simulink model "generic_IsaacV3"  (R2015a)
settings: Solver=ode3  StartTime=0.0  StopTime=inf  FixedStep=0.001  RelTol=1e-3
values from neighbouring files (symbols this model uses):
  coast_domain = 0.1    [LoadVar.m]
  DifferentialFactor = 0.5    [LoadVar.m]
  g = 9.81    [LoadVar.m]
  GearRatio = 10.364    [LoadVar.m]
  Gr = 10.32    [LoadVar.m]
  Lf = 0.78    [LoadVar.m]
  Lr = 0.745    [LoadVar.m]
  M = 265    [LoadVar.m]
  max_coast_Nm = 0    [LoadVar.m]
  MaxSteeringAngle = 24.635    [LoadVar.m]
  mu_max = 1.5    [LoadVar.m]
  ped_max_limiet = 1    [LoadVar.m]
  pedal_position_maxacc = 0.9    [LoadVar.m]
  Reff = 0.2325    [LoadVar.m]
  regen_activation_kph = 15    [LoadVar.m]
  slewbreak_domain = 0.15    [LoadVar.m]
  Sr = 0.6    [LoadVar.m]
  T_max_Nm = 40    [LoadVar.m]
  T_min_Nm = -15    [LoadVar.m]
  TireRadius = 0.4572/2    (= 0.2286)    [LoadVar.m]
  Tmax = 40    [LoadVar.m]
  TrackLength = 1.534    [LoadVar.m]
  TrackWidth = 1.200    (= 1.2)    [LoadVar.m]
libraries: CarMaker4SL x21, simulink x7
(part 2 of 3)

== system generic_IsaacV3/CarMaker/SignalOut/CreateBus PTC MotorOut0 ==
  In : Inport
  Bus Creator : BusCreator  Inputs=3
  BusCreator : BusCreator  Inputs=3
  Demux : Demux  Outputs=3
  "Load_mode_Not set " : Constant  Value=-99999
  "Speed_mode_notSet " : Constant  Value=-99999
  Out : Outport
  wires:
  BusCreator/1 -> Out/1
  Demux/3 -> BusCreator/3  "PTC MotorOut0 rotv_trg"
  Demux/2 -> BusCreator/2  "PTC MotorOut0 Trq_trg"
  Demux/1 -> BusCreator/1  "PTC MotorOut0 Load"
  Bus Creator/1 -> Demux/1
  In/1 -> Bus Creator/2  "Torque_mode"
  "Load_mode_Not set "/1 -> Bus Creator/1
  "Speed_mode_notSet "/1 -> Bus Creator/3

== system generic_IsaacV3/CarMaker/SignalOut/CreateBus PTC MotorOut1 ==
  In : Inport
  Bus Creator : BusCreator  Inputs=3
  BusCreator : BusCreator  Inputs=3
  Demux : Demux  Outputs=3
  "Load_mode_Not set " : Constant  Value=-99999
  "Speed_mode_notSet " : Constant  Value=-99999
  Out : Outport
  wires:
  BusCreator/1 -> Out/1
  Demux/2 -> BusCreator/2  "PTC MotorOut1 Trq_trg"
  Demux/3 -> BusCreator/3  "PTC MotorOut1 rotv_trg"
  Demux/1 -> BusCreator/1  "PTC MotorOut1 Load"
  "Load_mode_Not set "/1 -> Bus Creator/1
  "Speed_mode_notSet "/1 -> Bus Creator/3
  Bus Creator/1 -> Demux/1
  In/1 -> Bus Creator/2

== system generic_IsaacV3/CarMaker/SignalOut/CreateBus PTC MotorOut2 ==
  In : Inport
  BusCreator : BusCreator  Inputs=3
  Demux : Demux  Outputs=3
  Out : Outport
  wires:
  In/1 -> Demux/1
  BusCreator/1 -> Out/1
  Demux/1 -> BusCreator/1  "PTC MotorOut2 Load"
  Demux/2 -> BusCreator/2  "PTC MotorOut2 Trq_trg"
  Demux/3 -> BusCreator/3  "PTC MotorOut2 rotv_trg"

== system generic_IsaacV3/CarMaker/SignalOut/CreateBus PTC MotorOut3 ==
  In : Inport
  BusCreator : BusCreator  Inputs=3
  Demux : Demux  Outputs=3
  Out : Outport
  wires:
  In/1 -> Demux/1
  BusCreator/1 -> Out/1
  Demux/1 -> BusCreator/1  "PTC MotorOut3 Load"
  Demux/2 -> BusCreator/2  "PTC MotorOut3 Trq_trg"
  Demux/3 -> BusCreator/3  "PTC MotorOut3 rotv_trg"

== system generic_IsaacV3/CarMaker/SignalOut/CreateBus PTC PwrSupplyOut ==
  In : Inport
  BusCreator : BusCreator  Inputs=1
  Demux : Demux  Outputs=1
  Out : Outport
  wires:
  In/1 -> Demux/1
  BusCreator/1 -> Out/1
  Demux/1 -> BusCreator/1  "PTC PwrSupplyOut Pwr_HV1toLV_trg"

== system generic_IsaacV3/CarMaker/SignalOut/CreateBus PTC WheelOut ==
  In : Inport
  BusCreator : BusCreator  Inputs=8
  Demux : Demux  Outputs=8
  Out : Outport
  wires:
  In/1 -> Demux/1
  BusCreator/1 -> Out/1
  Demux/1 -> BusCreator/1  "PTC WheelOut_FL Trq_BrakeReg"
  Demux/2 -> BusCreator/2  "PTC WheelOut_FL Trq_BrakeReg_max"
  Demux/3 -> BusCreator/3  "PTC WheelOut_FR Trq_BrakeReg"
  Demux/4 -> BusCreator/4  "PTC WheelOut_FR Trq_BrakeReg_max"
  Demux/5 -> BusCreator/5  "PTC WheelOut_RL Trq_BrakeReg"
  Demux/6 -> BusCreator/6  "PTC WheelOut_RL Trq_BrakeReg_max"
  Demux/7 -> BusCreator/7  "PTC WheelOut_RR Trq_BrakeReg"
  Demux/8 -> BusCreator/8  "PTC WheelOut_RR Trq_BrakeReg_max"

== system generic_IsaacV3/CarMaker/SignalOut/PTC ==
  Constant2 : Constant
  Ground : Ground
  Mode_EngineDrive : Constant  Value=4
  Mux : Mux
  OperState_Driving : Constant  Value=4
  PTC MiscOut : Outport
  wires:
  Mux/1 -> PTC MiscOut/1
  OperState_Driving/1 -> Mux/1
  Ground/1 -> Mux/2  "OperationError"
  Mode_EngineDrive/1 -> Mux/3
  Constant2/1 -> Mux/4  "Ignition"

== system generic_IsaacV3/CarMaker/SignalOut/PTControl_Out ==
  PTC MiscOut : Inport
  PTC EngineOut : Inport  Port=2
  PTC ISGOut : Inport  Port=3
  PTC MotorOut0 : Inport  Port=4
  PTC MotorOut1 : Inport  Port=5
  PTC MotorOut2 : Inport  Port=6
  PTC MotorOut3 : Inport  Port=7
  PTC ClutchOut : Inport  Port=8
  PTC GearBoxOut : Inport  Port=9
  PTC GearBoxM_Out0 : Inport  Port=10
  PTC GearBoxM_Out1 : Inport  Port=11
  PTC GearBoxM_Out2 : Inport  Port=12
  PTC GearBoxM_Out3 : Inport  Port=13
  PTC PwrSupplyOut : Inport  Port=14
  PTC WheelOut : Inport  Port=15
  PTControl_Out : S-Function  FunctionName=cm_ptcontrol_out
  wires:
  PTC MiscOut/1 -> PTControl_Out/1
  PTC EngineOut/1 -> PTControl_Out/2
  PTC ISGOut/1 -> PTControl_Out/3
  PTC MotorOut0/1 -> PTControl_Out/4
  PTC MotorOut1/1 -> PTControl_Out/5
  PTC MotorOut2/1 -> PTControl_Out/6
  PTC MotorOut3/1 -> PTControl_Out/7
  PTC ClutchOut/1 -> PTControl_Out/8
  PTC GearBoxOut/1 -> PTControl_Out/9
  PTC GearBoxM_Out0/1 -> PTControl_Out/10
  PTC GearBoxM_Out1/1 -> PTControl_Out/11
  PTC GearBoxM_Out2/1 -> PTControl_Out/12
  PTC GearBoxM_Out3/1 -> PTControl_Out/13
  PTC PwrSupplyOut/1 -> PTControl_Out/14
  PTC WheelOut/1 -> PTControl_Out/15

== system generic_IsaacV3/CarMaker/TorqueVectoring/PI_CONTROLLER1 ==
  YawRate-Error : Inport
  Vzwp : Inport  Port=2
  Clamping circuit : Subsystem
  Constant : Constant  DisableCoverage=on  Value=0  OutDataTypeStr=Inherit: Inherit via back propagation  PreserveConstantTs=on
  Discrete-Time Integrator : DiscreteIntegrator  InitialConditionSetting=State (most efficient)  SampleTime=0.001  LimitOutput=on  UpperSaturationLimit=100  LowerSaturationLimit=-100
  Gain1 : Gain  Gain=1/10
  Gain2 : Gain  Gain=1/1000
  I : Product  RndMeth=Zero
  Lookup Table IifV : Lookup  InputValues=[-1 1 3 5 7 8 10 12 13 15 18 22 26 30 35 40]  Table=[50352886.7892156 50352886.7892156 5589135.45551528 1921428.35851846 975393.735493402 705695.225360316 447460.758905211 279243.629097448 236454.771525978 158654.332416002 94344.5016145154 48661.6461191947 26632.8595225856 13884.3621478696 5589.69756030357 1773.78141835761]
  Lookup Table PifV : Lookup  InputValues=[-1 1 3 5 7 8 10 12 13 15 18 22 26 30 35 40]  Table=[34635.2718980569 34635.2718980569 11590.7926431014 6627.38536761836 4783.12358808128 3932.42492202412 3196.93917901615 2407.06272090184 2253.13792386493 1777.83703218778 1346.39413645714 954.27715290151 744.973517942164 573.513734145603 406.894553185122 261.731683767634]
  P : Product  RndMeth=Zero
  Saturation : Saturate  UpperLimit=500  LowerLimit=-500
  Sum1 : Sum
  Switch : Switch  Criteria=u2 > Threshold  SaturateOnIntegerOverflow=on  InputSameDT=on
  PI_out : Outport
  wires:
  Lookup Table PifV/1 -> Gain1/1  "P_actie"
  Lookup Table IifV/1 -> Gain2/1  "I_actie"
  P/1 -> Sum1/1
  Sum1/1 -> Clamping circuit/1(preSat), Saturation/1  "Gewenste waarde"
  I/1 -> Clamping circuit/2(preIntegrator), Switch/3
  Saturation/1 -> PI_out/1  "Output controller"
  Gain1/1 -> P/1
  YawRate-Error/1 -> P/2, I/1  "Error"
  Vzwp/1 -> Lookup Table PifV/1, Lookup Table IifV/1  "V"
  Gain2/1 -> I/2
  Clamping circuit/1(Clamp) -> Switch/2
  Constant/1 -> Switch/1
  Switch/1 -> Discrete-Time Integrator/1
  Discrete-Time Integrator/1 -> Sum1/2

== system generic_IsaacV3/CarMaker/TorqueVectoring/Post-processor ==
  ax : Inport
  ay : Inport  Port=2
  mu_max : Inport  Port=3
  Vzwp : Inport  Port=4
  Mz : Inport  Port=5
  Tgevraagd : Inport  Port=6
  Fysische beperkingen : Subsystem
  Reff : Gain  Gain=Reff
  Reff1 : Gain  Gain=Reff
  Saturation : Saturate  UpperLimit=Gr*Tmax*mu_max  LowerLimit=-Gr*Tmax*mu_max
  Saturation1 : Saturate  UpperLimit=Gr*Tmax*mu_max  LowerLimit=-Gr*Tmax*mu_max
  "Slip-controle " : MATLAB Function  TreatAsAtomicUnit=on
  Sqrt : Sqrt  SaturateOnIntegerOverflow=on
  Sqrt1 : Sqrt  SaturateOnIntegerOverflow=on
  Sum : Sum  Inputs=|++
  Sum1 : Sum  Inputs=|++
  Trl : Outport
  Trr : Outport  Port=2
  Wf : Outport  Port=3
  Wr : Outport  Port=4
  wires:
  Fysische beperkingen/2(Trr) -> Trr/1
  Fysische beperkingen/1(Trl) -> Trl/1
  Saturation1/1 -> Fysische beperkingen/2(Trr_maxB)
  Saturation/1 -> Fysische beperkingen/1(Trl_maxB)
  Tgevraagd/1 -> Fysische beperkingen/4(Tgevraagd)
  Mz/1 -> Fysische beperkingen/3(Mz)
  mu_max/1 -> "Slip-controle "/3(mu_max)
  Vzwp/1 -> "Slip-controle "/4(Vzwp)
  ax/1 -> "Slip-controle "/1(ax)
  ay/1 -> "Slip-controle "/2(ay)
  "Slip-controle "/1(A) -> Sum/1
  "Slip-controle "/3(C) -> Sum1/1
  "Slip-controle "/2(B) -> Sum/2
  "Slip-controle "/4(D) -> Sum1/2
  Sum/1 -> Sqrt/1
  Sum1/1 -> Sqrt1/1
  Sqrt1/1 -> Reff1/1
  Sqrt/1 -> Reff/1
  Reff/1 -> Saturation/1
  Reff1/1 -> Saturation1/1
  "Slip-controle "/6(Wr) -> Wr/1
  "Slip-controle "/5(Wf) -> Wf/1

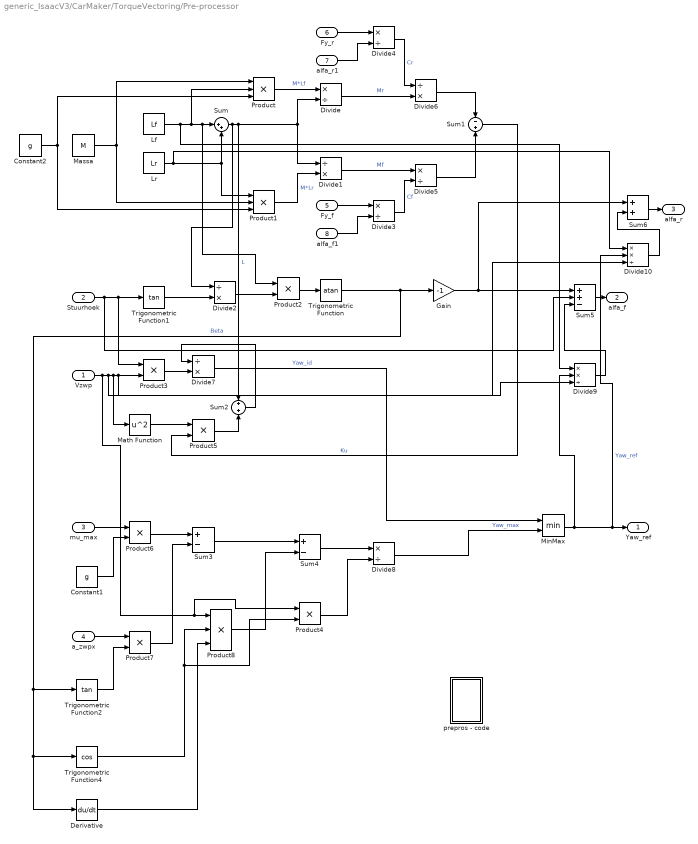
== system generic_IsaacV3/CarMaker/TorqueVectoring/Pre-processor ==
  Vzwp : Inport
  Stuurhoek : Inport  Port=2
  mu_max : Inport  Port=3
  a_zwpx : Inport  Port=4
  Fy_f : Inport  Port=5
  Fy_r : Inport  Port=6
  alfa_r1 : Inport  Port=7
  alfa_f1 : Inport  Port=8
  Constant1 : Constant  Value=g
  Constant2 : Constant  Value=g
  Derivative : Derivative
  Divide{,3..5,8} (5 alike) : Product  Inputs=*/
  Divide{1..2,6..7} (4 alike) : Product  Inputs=/*
  Divide10 : Product  Inputs=**/
  Divide9 : Product  Inputs=**/
  Gain : Gain  Gain=-1
  Lf : Constant  Value=Lf
  Lr : Constant  Value=Lr
  Massa : Constant  Value=M
  Math Function : Math  Operator=square  SaturateOnIntegerOverflow=on
  MinMax : MinMax  Inputs=2
  Product : Product  Inputs=3
  Product1 : Product  Inputs=3
  Product{2..7} (6 alike) : Product
  Product8 : Product  Inputs=3
  Sum : Sum  Inputs=|++
  Sum1 : Sum  Inputs=-+
  Sum2 : Sum
  Sum3 : Sum  Inputs=+-
  Sum4 : Sum  Inputs=+-
  Sum5 : Sum  Inputs=++-
  Sum6 : Sum
  Trigonometric Function : Trigonometry  Operator=atan
  Trigonometric Function1 : Trigonometry  Operator=tan
  Trigonometric Function2 : Trigonometry  Operator=tan
  Trigonometric Function4 : Trigonometry  Operator=cos
  prepros - code : Subsystem
  Yaw_ref : Outport
  alfa_f : Outport  Port=2
  alfa_r : Outport  Port=3
  wires:
  Product8/1 -> Sum4/2
  Product4/1 -> Divide8/2
  Derivative/1 -> Product8/3
  MinMax/1 -> Divide9/2, Divide10/2, Yaw_ref/1  "Yaw_ref"
  Divide8/1 -> MinMax/2  "Yaw_max"
  Sum4/1 -> Divide8/1
  Fy_r/1 -> Divide4/1
  Divide4/1 -> Divide6/1  "Cr"
  Divide6/1 -> Sum1/1
  Trigonometric Function1/1 -> Divide2/2
  Divide1/1 -> Divide5/1  "Mf"
  Divide2/1 -> Product2/2
  alfa_f1/1 -> Divide3/2
  Divide/1 -> Divide6/2  "Mr"
  Trigonometric Function/1 -> Gain/1, Trigonometric Function2/1, Derivative/1, Trigonometric Function4/1  "Beta"
  alfa_r1/1 -> Divide4/2
  Product1/1 -> Divide1/2  "M*Lr"
  Lf/1 -> Divide9/1, Product/2, Product2/1, Sum/1
  Product2/1 -> Trigonometric Function/1
  Divide3/1 -> Divide5/2  "Cf"
  Massa/1 -> Product/1, Product1/2
  Product/1 -> Divide/1  "M*Lf"
  Sum/1 -> Divide/2, Divide1/1, Sum2/1, Divide2/1  "L"
  Lr/1 -> Divide10/1, Product1/1, Sum/2
  Math Function/1 -> Product5/1
  mu_max/1 -> Product6/1
  Trigonometric Function4/1 -> Product4/2, Product8/2
  Product5/1 -> Sum2/2
  Product6/1 -> Sum3/1
  Constant1/1 -> Product6/2
  Sum1/1 -> Product5/2  "Ku"
  Divide7/1 -> MinMax/1  "Yaw_id"
  Product7/1 -> Sum3/2
  Sum3/1 -> Sum4/1
  Divide5/1 -> Sum1/2
  Sum2/1 -> Divide7/1
  Vzwp/1 -> Product4/1, Product8/1, Divide9/3, Math Function/1, Divide10/3, Product3/2
  Trigonometric Function2/1 -> Product7/2
  a_zwpx/1 -> Product7/1
  Product3/1 -> Divide7/2
  Gain/1 -> Sum6/1, Sum5/1
  Divide9/1 -> Sum5/3
  Sum5/1 -> alfa_f/1
  Divide10/1 -> Sum6/2
  Sum6/1 -> alfa_r/1
  Constant2/1 -> Product1/3, Product/3
  Fy_f/1 -> Divide3/1
  Stuurhoek/1 -> Sum5/2, Product3/1, Trigonometric Function1/1

== system generic_IsaacV3/CarMaker/Vehicle Sensors/PreProcessor ==
  SensorBus : Inport
  Bus Creator : BusCreator  Inputs=5
  Bus Selector : BusSelector  OutputSignals=Read_WheelspeedFL_rad/s,Read_WheelspeedFR_rad/s,Read_WheelspeedRL_rad/s,Read_WheelspeedRR_rad/s
  MATLAB Function : MATLAB Function  TreatAsAtomicUnit=on
  SensorBusOut : Outport
  wires:
  SensorBus/1 -> Bus Creator/5, Bus Selector/1
  Bus Selector/1 -> MATLAB Function/1(speedfl)  "<Read_WheelspeedFL_rad/s>"
  Bus Selector/2 -> MATLAB Function/2(speedfr)  "<Read_WheelspeedFR_rad/s>"
  Bus Selector/3 -> MATLAB Function/3(speedrl)  "<Read_WheelspeedRL_rad/s>"
  Bus Selector/4 -> MATLAB Function/4(speedrr)  "<Read_WheelspeedRR_rad/s>"
  MATLAB Function/1(slip_ratio_gem) -> Bus Creator/1  "SR_gem"
  MATLAB Function/2(vehicle_speed_mps) -> Bus Creator/2  "Vehicle_velocity_mps"
  MATLAB Function/3(slip_ratio_RL) -> Bus Creator/3  "SR_RL"
  MATLAB Function/4(slip_ratio_RR) -> Bus Creator/4  "SR_RR"
  Bus Creator/1 -> SensorBusOut/1

== system generic_IsaacV3/CarMaker/Vehicle Sensors/SensorIn Plots ==
  SensorBus : Inport
  Bus Selector : BusSelector  OutputSignals=SensorBus.Read_ElecMotorPowerRL_kW,SensorBus.Read_ElecMotorPowerRR_kW
  Bus Selector1 : BusSelector  OutputSignals=SensorBus.Read_WheelspeedFL_rad/s,SensorBus.Read_WheelspeedFR_rad/s,SensorBus.Read_WheelspeedRL_rad/s,SensorBus.Read_WheelspeedRR_rad/s
  Bus Selector2 : BusSelector  OutputSignals=SensorBus.Read_Steering_angle_rad
  Bus Selector3 : BusSelector  OutputSignals=SR_RL,SR_RR
  Gain{,1..3} (4 alike) : Gain  Gain=60/(2*pi)
  Gain4 : Gain  Gain=360/(2*pi)
  MotorPower_kW : Scope  NumInputPorts=2
      settings: YMin=-40~-20  YMax=65~65  SaveName=ScopeData9
  Rear Slip Ratio : Scope  NumInputPorts=2
      settings: YMin=-0.5~-0.5  YMax=1~1  SaveName=ScopeData19
  SteeringAngle_degrees : Scope
      settings: YMin=-2  YMax=2  SaveName=ScopeData15
  Wheelspeed_RPM : Scope  NumInputPorts=4
      settings: YMin=-100~-100~-100~-100  YMax=2400~2400~2400~2400  SaveName=ScopeData12
  wires:
  SensorBus/1 -> Bus Selector3/1, Bus Selector2/1, Bus Selector1/1, Bus Selector/1
  Bus Selector/1 -> MotorPower_kW/1  "<Read_ElecMotorPowerRL_kW>"
  Bus Selector/2 -> MotorPower_kW/2  "<Read_ElecMotorPowerRR_kW>"
  Gain1/1 -> Wheelspeed_RPM/2  "Read_WheelspeedFR_RPM"
  Gain/1 -> Wheelspeed_RPM/1  "Read_WheelspeedFL_RPM"
  Gain2/1 -> Wheelspeed_RPM/3  "Read_WheelspeedRL_RPM"
  Gain3/1 -> Wheelspeed_RPM/4  "Read_WheelspeedRR_RPM"
  Bus Selector1/4 -> Gain3/1  "<Read_WheelspeedRR_rad/s>"
  Bus Selector1/3 -> Gain2/1  "<Read_WheelspeedRL_rad/s>"
  Bus Selector1/2 -> Gain1/1  "<Read_WheelspeedFR_rad/s>"
  Bus Selector1/1 -> Gain/1  "<Read_WheelspeedFL_rad/s>"
  Bus Selector2/1 -> Gain4/1  "<Read_Steering_angle_rad>"
  Bus Selector3/1 -> Rear Slip Ratio/1  "<SR_RL>"
  Bus Selector3/2 -> Rear Slip Ratio/2  "<SR_RR>"
  Gain4/1 -> SteeringAngle_degrees/1  "Read_SteeringAngle_degrees"

== system generic_IsaacV3/CarMaker/VehicleControl/CreateBus Vhcl.Misc ==
  In1 : Inport
  Bus Creator5 : BusCreator  Inputs=11
  Demux5 : Demux  Outputs=11
  Out1 : Outport
  wires:
  Demux5/11 -> Bus Creator5/11  "Vhcl Wind_vel_0 z"
  Demux5/10 -> Bus Creator5/10  "Vhcl Wind_vel_0 y"
  Demux5/9 -> Bus Creator5/9  "Vhcl Wind_vel_0 x"
  Demux5/8 -> Bus Creator5/8  "Vhcl DL2BdyEng y"
  Demux5/7 -> Bus Creator5/7  "Vhcl DL2BdyEng x"
  Demux5/6 -> Bus Creator5/6  "Vhcl TrqDL2Bdy1B z"
  Demux5/5 -> Bus Creator5/5  "Vhcl TrqDL2Bdy1B y"
  Demux5/4 -> Bus Creator5/4  "Vhcl TrqDL2Bdy1B x"
  Demux5/3 -> Bus Creator5/3  "Vhcl Trq_DL2Bdy1 z"
  In1/1 -> Demux5/1
  Bus Creator5/1 -> Out1/1
  Demux5/2 -> Bus Creator5/2  "Vhcl Trq_DL2Bdy1 y"
  Demux5/1 -> Bus Creator5/1  "Vhcl Trq_DL2Bdy1 x"

== system generic_IsaacV3/CarMaker/VehicleControl/CreateBus Vhcl.Wheel.In ==
  In1 : Inport
  Bus Creator1 : BusCreator  Inputs=12
  Demux1 : Demux  Outputs=12
  Scope{,1..5} (6 alike) : Scope
      Scope1 settings: YMin=-400  YMax=400  SaveName=ScopeData2
      Scope2 settings: YMin=-10  YMax=400  SaveName=ScopeData3
      Scope3 settings: YMin=-400  YMax=400  SaveName=ScopeData4
      Scope4 settings: YMin=-400  YMax=400  SaveName=ScopeData5
      Scope5 settings: SaveName=ScopeData6
  Out1 : Outport
  wires:
  Demux1/12 -> Scope2/1, Bus Creator1/12  "Vhcl Wheel RR rotv"
  Demux1/11 -> Scope1/1, Bus Creator1/11  "Vhcl Wheel RR Trq_DL2WC"
  Demux1/10 -> Scope/1, Bus Creator1/10  "Vhcl Wheel RR Trq_B2WC"
  Demux1/9 -> Scope3/1, Bus Creator1/9  "Vhcl Wheel RL rotv"
  Demux1/8 -> Scope4/1, Bus Creator1/8  "Vhcl Wheel RL Trq_DL2WC"
  Demux1/7 -> Scope5/1, Bus Creator1/7  "Vhcl Wheel RL Trq_B2WC"
  Demux1/6 -> Bus Creator1/6  "Vhcl Wheel FR rotv"
  Demux1/5 -> Bus Creator1/5  "Vhcl Wheel FR Trq_DL2WC"
  Demux1/4 -> Bus Creator1/4  "Vhcl Wheel FR Trq_B2WC"
  Demux1/3 -> Bus Creator1/3  "Vhcl Wheel FL rotv"
  In1/1 -> Demux1/1
  Bus Creator1/1 -> Out1/1
  Demux1/2 -> Bus Creator1/2  "Vhcl Wheel FL Trq_DL2WC"
  Demux1/1 -> Bus Creator1/1  "Vhcl Wheel FL Trq_B2WC"

== system generic_IsaacV3/CarMaker/VehicleControl/CreateBus VhclCtrl ==
  In : Inport
  BusCreator : BusCreator  Inputs=29
  Demux : Demux  Outputs=29
  Out : Outport
  wires:
  In/1 -> Demux/1
  BusCreator/1 -> Out/1
  Demux/1 -> BusCreator/1  "VhclCtrl SST"
  Demux/2 -> BusCreator/2  "VhclCtrl Key"
  Demux/3 -> BusCreator/3  "VhclCtrl UserSignal0"
  Demux/4 -> BusCreator/4  "VhclCtrl UserSignal1"
  Demux/5 -> BusCreator/5  "VhclCtrl UserSignal2"
  Demux/6 -> BusCreator/6  "VhclCtrl UserSignal3"
  Demux/7 -> BusCreator/7  "VhclCtrl UserSignal4"
  Demux/8 -> BusCreator/8  "VhclCtrl GearNo"
  Demux/9 -> BusCreator/9  "VhclCtrl SelectorCtrl"
  Demux/10 -> BusCreator/10  "VhclCtrl Brake"
  Demux/11 -> BusCreator/11  "VhclCtrl BrakePark"
  Demux/12 -> BusCreator/12  "VhclCtrl Clutch"
  Demux/13 -> BusCreator/13  "VhclCtrl Gas"
  Demux/14 -> BusCreator/14  "VhclCtrl Steering Ang"
  Demux/15 -> BusCreator/15  "VhclCtrl Steering AngVel"
  Demux/16 -> BusCreator/16  "VhclCtrl Steering AngAcc"
  Demux/17 -> BusCreator/17  "VhclCtrl Steering Trq"
  Demux/18 -> BusCreator/18  "VhclCtrl Lights LowBeam"
  Demux/19 -> BusCreator/19  "VhclCtrl Lights HighBeam"
  Demux/20 -> BusCreator/20  "VhclCtrl Lights Daytime"
  Demux/21 -> BusCreator/21  "VhclCtrl Lights ParkL"
  Demux/22 -> BusCreator/22  "VhclCtrl Lights ParkR"
  Demux/23 -> BusCreator/23  "VhclCtrl Lights IndL"
  Demux/24 -> BusCreator/24  "VhclCtrl Lights IndR"
  Demux/25 -> BusCreator/25  "VhclCtrl Lights FogFrontL"
  Demux/26 -> BusCreator/26  "VhclCtrl Lights FogFrontR"
  Demux/27 -> BusCreator/27  "VhclCtrl Lights FogRear"
  Demux/28 -> BusCreator/28  "VhclCtrl Lights Brake"
  Demux/29 -> BusCreator/29  "VhclCtrl Lights Reverse"

== system generic_IsaacV3/CarMaker/VehicleControl/CreateBus VhclCtrl.PT ==
  In1 : Inport
  BusCreator : BusCreator  Inputs=11
  Demux : Demux  Outputs=11
  Out1 : Outport
  wires:
  In1/1 -> Demux/1
  BusCreator/1 -> Out1/1
  Demux/1 -> BusCreator/1  "VhclCtrl SST"
  Demux/2 -> BusCreator/2  "VhclCtrl Key"
  Demux/3 -> BusCreator/3  "VhclCtrl UserSignal0"
  Demux/4 -> BusCreator/4  "VhclCtrl UserSignal1"
  Demux/5 -> BusCreator/5  "VhclCtrl UserSignal2"
  Demux/6 -> BusCreator/6  "VhclCtrl UserSignal3"
  Demux/7 -> BusCreator/7  "VhclCtrl UserSignal4"
  Demux/8 -> BusCreator/8  "VhclCtrl GearNo"
  Demux/9 -> BusCreator/9  "VhclCtrl SelectorCtrl"
  Demux/10 -> BusCreator/10  "VhclCtrl Clutch"
  Demux/11 -> BusCreator/11  "VhclCtrl Gas"

== system generic_IsaacV3/CarMaker/VehicleControl/CreateBus VhclCtrl.Steering ==
  In1 : Inport
  Bus Creator : BusCreator  Inputs=5
  Demux : Demux  Outputs=5
  Out1 : Outport
  wires:
  In1/1 -> Demux/1
  Bus Creator/1 -> Out1/1
  Demux/1 -> Bus Creator/1  "VhclCtrl Steering Ang"
  Demux/5 -> Bus Creator/5  "VhclCtrl Steering ByTrq"
  Demux/3 -> Bus Creator/3  "VhclCtrl Steering AngAcc"
  Demux/2 -> Bus Creator/2  "VhclCtrl Steering AngVel"
  Demux/4 -> Bus Creator/4  "VhclCtrl Steering Trq"

== system generic_IsaacV3/CarMaker/IPG Vehicle/Brake/CreateBus Vhcl.Wheel.PT ==
  In : Inport
  BusCreator : BusCreator  Inputs=16
  Demux : Demux  Outputs=16
  Out : Outport
  wires:
  Demux/16 -> BusCreator/16  "Vhcl Wheel RR WhlBearing"
  Demux/15 -> BusCreator/15  "Vhcl Wheel RR Trq_T2W"
  Demux/14 -> BusCreator/14  "Vhcl Wheel RR Trq_BrakeReg_trg"
  Demux/13 -> BusCreator/13  "Vhcl Wheel RR Trq_Brake"
  Demux/12 -> BusCreator/12  "Vhcl Wheel RL WhlBearing"
  Demux/11 -> BusCreator/11  "Vhcl Wheel RL Trq_T2W"
  Demux/10 -> BusCreator/10  "Vhcl Wheel RL Trq_BrakeReg_trg"
  Demux/9 -> BusCreator/9  "Vhcl Wheel RL Trq_Brake"
  Demux/8 -> BusCreator/8  "Vhcl Wheel FR WhlBearing"
  Demux/7 -> BusCreator/7  "Vhcl Wheel FR Trq_T2W"
  Demux/6 -> BusCreator/6  "Vhcl Wheel FR Trq_BrakeReg_trg"
  Demux/5 -> BusCreator/5  "Vhcl Wheel FR Trq_Brake"
  Demux/4 -> BusCreator/4  "Vhcl Wheel FL WhlBearing"
  Demux/3 -> BusCreator/3  "Vhcl Wheel FL Trq_T2W"
  Demux/2 -> BusCreator/2  "Vhcl Wheel FL Trq_BrakeReg_trg"
  Demux/1 -> BusCreator/1  "Vhcl Wheel FL Trq_Brake"
  BusCreator/1 -> Out/1
  In/1 -> Demux/1

== system generic_IsaacV3/CarMaker/IPG Vehicle/CarAndTrailer/CarAndTrailerUpd ==
  Sync_In : Inport
  Vhcl.Steering : Inport  Port=2
  Vhcl.Motion : Inport  Port=3
  Vhcl.PoI : Inport  Port=4
  Vhcl.Wheel.FL : Inport  Port=5
  Vhcl.Wheel.FR : Inport  Port=6
  Vhcl.Wheel.RL : Inport  Port=7
  Vhcl.Wheel.RR : Inport  Port=8
  Car.Hitch.FrcTrq : Inport  Port=9
  Vhcl.Fr1A : Inport  Port=10
  CarAndTrailerUpd : S-Function  FunctionName=CM_Sfun  Parameters='CarAndTrUpd'
  CreateBus Brake.IF.In : Subsystem
  Sync_Out : Outport
  Brake.IF.In : Outport  Port=2
  wires:
  Vhcl.Fr1A/1 -> CarAndTrailerUpd/10  "user vehicle only"
  Vhcl.Steering/1 -> CarAndTrailerUpd/2
  Vhcl.Motion/1 -> CarAndTrailerUpd/3
  Vhcl.PoI/1 -> CarAndTrailerUpd/4
  Vhcl.Wheel.FL/1 -> CarAndTrailerUpd/5
  Vhcl.Wheel.FR/1 -> CarAndTrailerUpd/6
  Car.Hitch.FrcTrq/1 -> CarAndTrailerUpd/9
  Vhcl.Wheel.RR/1 -> CarAndTrailerUpd/8
  Vhcl.Wheel.RL/1 -> CarAndTrailerUpd/7
  CarAndTrailerUpd/2 -> CreateBus Brake.IF.In/1(In)
  CreateBus Brake.IF.In/1(Out) -> Brake.IF.In/1
  CarAndTrailerUpd/1 -> Sync_Out/1
  Sync_In/1 -> CarAndTrailerUpd/1

== system generic_IsaacV3/CarMaker/IPG Vehicle/CarAndTrailer/Forces ==
  Sync_In : Inport
  TireFL_In : Inport  Port=2
  TireFR_In : Inport  Port=3
  TireRL_In : Inport  Port=4
  TireRR_In : Inport  Port=5
  lSpring : Inport  Port=6
  vDamp : Inport  Port=7
  lStabi : Inport  Port=8
  lBuf : Inport  Port=9
  External Suspension Forces : Subsystem
  Tires : Subsystem
  Vehicle Forces : Subsystem
  Sync_Out : Outport
  Car.Virtual : Outport  Port=2
  Car.Aero : Outport  Port=3
  Car.Load : Outport  Port=4
  TireFL_Out : Outport  Port=5
  TireFR_Out : Outport  Port=6
  TireRL_Out : Outport  Port=7
  TireRR_Out : Outport  Port=8
  FSpring : Outport  Port=9
  FDamp : Outport  Port=10
  FStabi : Outport  Port=11
  FBuf : Outport  Port=12
  wires:
  External Suspension Forces/4(FBuf) -> FBuf/1
  lBuf/1 -> External Suspension Forces/5(lBuf)
  Tires/4(TireFL_Out) -> TireRR_Out/1
  Tires/3(TireRR_Out) -> TireRL_Out/1
  Tires/2(TireRL_Out) -> TireFR_Out/1
  Tires/1(TireFR_Out) -> TireFL_Out/1
  TireRR_In/1 -> Tires/5(TireFL_In)
  TireRL_In/1 -> Tires/4(TireRR_In)
  TireFR_In/1 -> Tires/3(TireRL_In)
  Sync_In/1 -> External Suspension Forces/1(Sync_In), Tires/1(Sync_In), Vehicle Forces/1(Sync_In)
  Vehicle Forces/1(Sync_Out) -> Sync_Out/1
  TireFL_In/1 -> Tires/2(TireFR_In)
  Vehicle Forces/2(Car.Virtual) -> Car.Virtual/1
  Vehicle Forces/3(Car.Aero) -> Car.Aero/1
  Vehicle Forces/4(Car.Load) -> Car.Load/1
  lSpring/1 -> External Suspension Forces/2(lSpring)
  External Suspension Forces/2(FDamp) -> FDamp/1
  vDamp/1 -> External Suspension Forces/3(vDamp)
  lStabi/1 -> External Suspension Forces/4(lStabi)
  External Suspension Forces/3(FStabi) -> FStabi/1
  External Suspension Forces/1(FSpring) -> FSpring/1

== system generic_IsaacV3/CarMaker/IPG Vehicle/CarAndTrailer/Kinematics ==
  Sync_In : Inport
  Steer.IF : Inport  Port=2
  Kinematics : S-Function  FunctionName=CM_Sfun  Parameters='Kinematics'
  Sync_Out : Outport
  TireFL_In : Outport  Port=2
  TireFR_In : Outport  Port=3
  TireRL_In : Outport  Port=4
  TireRR_In : Outport  Port=5
  lSpring : Outport  Port=6
  vDamp : Outport  Port=7
  lStabi : Outport  Port=8
  lBuf : Outport  Port=9
  wires:
  Kinematics/9 -> lBuf/1
  Kinematics/8 -> lStabi/1
  Kinematics/2 -> TireFL_In/1
  Kinematics/3 -> TireFR_In/1
  Kinematics/4 -> TireRL_In/1
  Kinematics/5 -> TireRR_In/1
  Kinematics/6 -> lSpring/1
  Kinematics/7 -> vDamp/1
  Sync_In/1 -> Kinematics/1
  Kinematics/1 -> Sync_Out/1
  Steer.IF/1 -> Kinematics/2

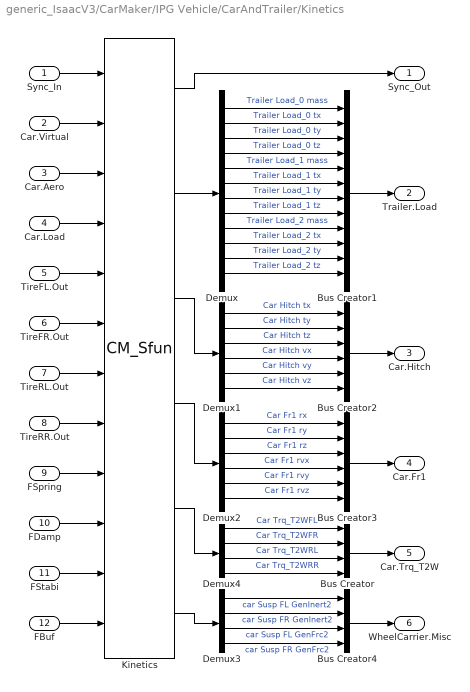
== system generic_IsaacV3/CarMaker/IPG Vehicle/CarAndTrailer/Kinetics ==
  Sync_In : Inport
  Car.Virtual : Inport  Port=2
  Car.Aero : Inport  Port=3
  Car.Load : Inport  Port=4
  TireFL.Out : Inport  Port=5
  TireFR.Out : Inport  Port=6
  TireRL.Out : Inport  Port=7
  TireRR.Out : Inport  Port=8
  FSpring : Inport  Port=9
  FDamp : Inport  Port=10
  FStabi : Inport  Port=11
  FBuf : Inport  Port=12
  Bus Creator : BusCreator
  Bus Creator1 : BusCreator  Inputs=12
  Bus Creator2 : BusCreator  Inputs=6
  Bus Creator3 : BusCreator  Inputs=6
  Bus Creator4 : BusCreator
  Demux : Demux  Outputs=12
  Demux1 : Demux  Outputs=6
  Demux2 : Demux  Outputs=6
  Demux3 : Demux
  Demux4 : Demux
  Kinetics : S-Function  FunctionName=CM_Sfun  Parameters='Kinetics'
  Sync_Out : Outport
  Trailer.Load : Outport  Port=2
  Car.Hitch : Outport  Port=3
  Car.Fr1 : Outport  Port=4
  Car.Trq_T2W : Outport  Port=5
  WheelCarrier.Misc : Outport  Port=6
  wires:
  FBuf/1 -> Kinetics/12
  Sync_In/1 -> Kinetics/1
  Kinetics/1 -> Sync_Out/1
  Car.Aero/1 -> Kinetics/3
  Car.Virtual/1 -> Kinetics/2
  Bus Creator1/1 -> Trailer.Load/1
  Demux/1 -> Bus Creator1/1  "Trailer Load_0 mass"
  Demux/2 -> Bus Creator1/2  "Trailer Load_0 tx"
  Demux/3 -> Bus Creator1/3  "Trailer Load_0 ty"
  Demux/4 -> Bus Creator1/4  "Trailer Load_0 tz"
  Kinetics/2 -> Demux/1
  Demux/5 -> Bus Creator1/5  "Trailer Load_1 mass"
  Demux/6 -> Bus Creator1/6  "Trailer Load_1 tx"
  Demux/7 -> Bus Creator1/7  "Trailer Load_1 ty"
  Demux/8 -> Bus Creator1/8  "Trailer Load_1 tz"
  Demux/9 -> Bus Creator1/9  "Trailer Load_2 mass"
  Demux/10 -> Bus Creator1/10  "Trailer Load_2 tx"
  Demux/11 -> Bus Creator1/11  "Trailer Load_2 ty"
  Demux/12 -> Bus Creator1/12  "Trailer Load_2 tz"
  Demux1/1 -> Bus Creator2/1  "Car Hitch tx"
  Demux1/2 -> Bus Creator2/2  "Car Hitch ty"
  Demux1/3 -> Bus Creator2/3  "Car Hitch tz"
  Demux1/4 -> Bus Creator2/4  "Car Hitch vx"
  Demux1/5 -> Bus Creator2/5  "Car Hitch vy"
  Demux1/6 -> Bus Creator2/6  "Car Hitch vz"
  Kinetics/3 -> Demux1/1
  Bus Creator2/1 -> Car.Hitch/1
  Demux2/1 -> Bus Creator3/1  "Car Fr1 rx"
  Demux2/2 -> Bus Creator3/2  "Car Fr1 ry"
  Demux2/3 -> Bus Creator3/3  "Car Fr1 rz"
  Demux2/4 -> Bus Creator3/4  "Car Fr1 rvx"
  Demux2/5 -> Bus Creator3/5  "Car Fr1 rvy"
  Demux2/6 -> Bus Creator3/6  "Car Fr1 rvz"
  Bus Creator3/1 -> Car.Fr1/1
  Kinetics/4 -> Demux2/1
  Car.Load/1 -> Kinetics/4
  Demux3/1 -> Bus Creator4/1  "car Susp FL GenInert2"
  Demux3/2 -> Bus Creator4/2  "car Susp FR GenInert2"
  Demux3/3 -> Bus Creator4/3  "car Susp FL GenFrc2"
  Demux3/4 -> Bus Creator4/4  "car Susp FR GenFrc2"
  Bus Creator4/1 -> WheelCarrier.Misc/1
  Bus Creator/1 -> Car.Trq_T2W/1
  Demux4/4 -> Bus Creator/4  "Car Trq_T2WRR"
  Demux4/3 -> Bus Creator/3  "Car Trq_T2WRL"
  Demux4/2 -> Bus Creator/2  "Car Trq_T2WFR"
  Demux4/1 -> Bus Creator/1  "Car Trq_T2WFL"
  TireFL.Out/1 -> Kinetics/5
  TireFR.Out/1 -> Kinetics/6
  TireRL.Out/1 -> Kinetics/7
  TireRR.Out/1 -> Kinetics/8
  FSpring/1 -> Kinetics/9
  FDamp/1 -> Kinetics/10
  FStabi/1 -> Kinetics/11
  Kinetics/6 -> Demux3/1
  Kinetics/5 -> Demux4/1

== system generic_IsaacV3/CarMaker/IPG Vehicle/CarAndTrailer/Steering ==
  note: When replacing the entire steering system,
      | be sure to add '-disablesteering' to the command line arguments
      | in the CarMaker Model Configuration block.
  Sync_In : Inport
  VhclCtrl.Steering : Inport  Port=2
  Bus Creator1 : BusCreator  Inputs=16
  Bus Creator2 : BusCreator
  Demux : Demux  Outputs=20
  Steering : S-Function  FunctionName=CM_Sfun  Parameters='Steering'
  Terminator : Terminator
  Sync_Out : Outport
  Steer.IF : Outport  Port=2
  wires:
  Bus Creator1/1 -> Steer.IF/1
  Steering/2 -> Demux/1
  Demux/8 -> Bus Creator1/8  "Steering IF AssistTrqPin"
  Demux/7 -> Bus Creator1/7  "Steering IF AssistTrqCol"
  Demux/6 -> Bus Creator1/6  "Steering IF AssistFrc"
  Demux/20 -> Bus Creator2/4  "Steering IF R Inert"
  Demux/17 -> Bus Creator2/1  "Steering IF L Frc"
  Demux/18 -> Bus Creator2/2  "Steering IF L Inert"
  Demux/19 -> Bus Creator2/3  "Steering IF R Frc"
  Bus Creator2/1 -> Terminator/1  "Steer IF (in)"
  Demux/16 -> Bus Creator1/16  "Steering IF R iSteer2q"
  Demux/9 -> Bus Creator1/9  "Steering IF L q"
  Demux/10 -> Bus Creator1/10  "Steering IF L qp"
  Demux/11 -> Bus Creator1/11  "Steering IF L qpp"
  Demux/12 -> Bus Creator1/12  "Steering IF L iSteer2q"
  Demux/13 -> Bus Creator1/13  "Steering IF R q"
  Demux/14 -> Bus Creator1/14  "Steering IF R qp"
  Demux/15 -> Bus Creator1/15  "Steering IF R qpp"
  VhclCtrl.Steering/1 -> Steering/2
  Steering/1 -> Sync_Out/1
  Sync_In/1 -> Steering/1
  Demux/1 -> Bus Creator1/1  "Steering IF Ang"
  Demux/2 -> Bus Creator1/2  "Steering IF AngVel"
  Demux/3 -> Bus Creator1/3  "Steering IF AngAcc"
  Demux/4 -> Bus Creator1/4  "Steering IF Trq"
  Demux/5 -> Bus Creator1/5  "Steering IF TrqStatic"

== system generic_IsaacV3/CarMaker/IPG Vehicle/CarAndTrailer/Trailer ==
  Sync_In : Inport
  Trailer.Load : Inport  Port=2
  Car.Hitch : Inport  Port=3
  Car.Fr1 : Inport  Port=4
  Car.Trq_T2W : Inport  Port=5
  WheelCarrier.Misc : Inport  Port=6
  CreateBus Car.Hitch.FrcTrq : Subsystem
  CreateBus Vhcl.Motion : Subsystem
  CreateBus Vhcl.PoI : Subsystem
  CreateBus Vhcl.Steering : Subsystem
  CreateBus Vhcl.Wheel.FL : Subsystem
  CreateBus Vhcl.Wheel.FR : Subsystem
  CreateBus Vhcl.Wheel.RL : Subsystem
  CreateBus Vhcl.Wheel.RR : Subsystem
  Trailer : S-Function  FunctionName=CM_Sfun  Parameters='Trailer'
  Sync_Out : Outport
  Vhcl.Steering : Outport  Port=2
  Vhcl.Motion : Outport  Port=3
  Vhcl.PoI : Outport  Port=4
  Vhcl.Wheel.FL : Outport  Port=5
  Vhcl.Wheel.FR : Outport  Port=6
  Vhcl.Wheel.RL : Outport  Port=7
  Vhcl.Wheel.RR : Outport  Port=8
  Car.Hitch.FrcTrq : Outport  Port=9
  wires:
  Trailer/2 -> CreateBus Vhcl.Steering/1(In1)
  CreateBus Vhcl.Steering/1(Out1) -> Vhcl.Steering/1
  Trailer/3 -> CreateBus Vhcl.Motion/1(In1)
  Trailer/4 -> CreateBus Vhcl.PoI/1(In1)
  Trailer/5 -> CreateBus Vhcl.Wheel.FL/1(In1)
  Trailer/6 -> CreateBus Vhcl.Wheel.FR/1(In1)
  Trailer/7 -> CreateBus Vhcl.Wheel.RL/1(In1)
  Trailer/9 -> CreateBus Car.Hitch.FrcTrq/1(In1)
  Trailer/8 -> CreateBus Vhcl.Wheel.RR/1(In1)
  CreateBus Vhcl.Wheel.RR/1(Out1) -> Vhcl.Wheel.RR/1  "Vhcl.Wheel.RR"
  CreateBus Vhcl.Wheel.RL/1(Out1) -> Vhcl.Wheel.RL/1  "Vhcl.Wheel.RL"
  CreateBus Vhcl.Wheel.FR/1(Out1) -> Vhcl.Wheel.FR/1  "Vhcl.Wheel.FR"
  CreateBus Vhcl.Wheel.FL/1(Out1) -> Vhcl.Wheel.FL/1  "Vhcl.Wheel.FL"
  CreateBus Vhcl.PoI/1(Out1) -> Vhcl.PoI/1
  CreateBus Vhcl.Motion/1(Out1) -> Vhcl.Motion/1
  Car.Trq_T2W/1 -> Trailer/5
  WheelCarrier.Misc/1 -> Trailer/6
  CreateBus Car.Hitch.FrcTrq/1(Car.Hitch.FrcTrq) -> Car.Hitch.FrcTrq/1
  Car.Fr1/1 -> Trailer/4
  Car.Hitch/1 -> Trailer/3
  Trailer.Load/1 -> Trailer/2
  Trailer/1 -> Sync_Out/1
  Sync_In/1 -> Trailer/1

== system generic_IsaacV3/CarMaker/TorqueVectoring/PI_CONTROLLER1/Clamping circuit ==
  preSat : Inport  DisableCoverage=on
  preIntegrator : Inport  DisableCoverage=on  Port=2
  AND : Logic  DisableCoverage=on
  DataTypeConv1 : DataTypeConversion  DisableCoverage=on  OutDataTypeStr=int8  SaturateOnIntegerOverflow=on  RndMeth=Zero  LockScale=on
  DataTypeConv2 : DataTypeConversion  DisableCoverage=on  OutDataTypeStr=int8  SaturateOnIntegerOverflow=on  RndMeth=Zero  LockScale=on
  DeadZone : DeadZone  DisableCoverage=on  LowerValue=-100  UpperValue=100  SaturateOnIntegerOverflow=on
  Equal : RelationalOperator  DisableCoverage=on  Operator===  InputSameDT=on
  Memory : Memory  DisableCoverage=on
  NotEqual : RelationalOperator  DisableCoverage=on  Operator=~=  InputSameDT=on
  SignDeltaU : Signum  DisableCoverage=on
  SignPreIntegrator : Signum  DisableCoverage=on
  ZeroGain : Gain  DisableCoverage=on  Gain=0  SaturateOnIntegerOverflow=on  OutDataTypeStr=Inherit: Same as input  ParamDataTypeStr=Inherit: Same as input
  Clamp : Outport  DisableCoverage=on
  wires:
  preSat/1 -> ZeroGain/1, DeadZone/1
  preIntegrator/1 -> SignPreIntegrator/1
  ZeroGain/1 -> NotEqual/1
  DeadZone/1 -> NotEqual/2, SignDeltaU/1
  SignDeltaU/1 -> DataTypeConv1/1
  DataTypeConv1/1 -> Equal/1
  SignPreIntegrator/1 -> DataTypeConv2/1
  DataTypeConv2/1 -> Equal/2
  NotEqual/1 -> AND/1
  Equal/1 -> AND/2
  AND/1 -> Memory/1
  Memory/1 -> Clamp/1

== system generic_IsaacV3/CarMaker/TorqueVectoring/Post-processor/Fysische beperkingen ==
  Trl_maxB : Inport
  Trr_maxB : Inport  Port=2
  Mz : Inport  Port=3
  Tgevraagd : Inport  Port=4
  Constant : Constant  Value=Gr
  Constant1 : Constant  Value=Reff
  Constant2 : Constant  Value=Sr
  Constant3 : Constant  Value=2
  Constant4 : Constant  Value=Gr
  Divide : Product  Inputs=/*
  Divide1 : Product  Inputs=*/
  Divide2 : Product  Inputs=*/
  Gain : Gain  Gain=-1
  Lineaire programmering code : Subsystem
  MinMax : MinMax  Inputs=2
  MinMax1 : MinMax  Inputs=2
  Product : Product
  Product1 : Product  Inputs=3
  Saturation1 : Saturate  UpperLimit=Tmax  LowerLimit=-Tmax
  Saturation2 : Saturate  UpperLimit=Tmax  LowerLimit=-Tmax
  Sum : Sum
  Sum1 : Sum
  Trl : Outport
  Trr : Outport  Port=2
  wires:
  Divide/1 -> Saturation2/1  "Trl_maxM"
  Trr_maxB/1 -> Divide1/1
  Constant2/1 -> Product1/1
  Product/1 -> Divide2/1
  Product1/1 -> Divide2/2
  Divide2/1 -> Gain/1, Sum/2  "Trl_2"
  Constant1/1 -> Product/1
  Sum1/1 -> Trr/1
  Constant4/1 -> Product1/2
  MinMax/1 -> Sum/1  "Trl_1"
  MinMax1/1 -> Sum1/1  "Trr_1"
  Constant/1 -> Divide/1, Divide1/2
  Trl_maxB/1 -> Divide/2
  Tgevraagd/1 -> MinMax1/1, MinMax/2
  Gain/1 -> Sum1/2  "Trr_2"
  Constant3/1 -> Product1/3
  Sum/1 -> Trl/1
  Mz/1 -> Product/2
  Divide1/1 -> Saturation1/1  "Trr_maxM"
  Saturation2/1 -> MinMax/1
  Saturation1/1 -> MinMax1/2

== system generic_IsaacV3/CarMaker/TorqueVectoring/Pre-processor/prepros - code ==
  Ground{,1..7} (8 alike) : Ground
  Pre-processor : MATLAB Function  TreatAsAtomicUnit=on
  Terminator : Terminator
  Terminator1 : Terminator
  Terminator2 : Terminator
  wires:
  Pre-processor/2(alfa_f) -> Terminator1/1
  Ground2/1 -> Pre-processor/6(Fy_r)
  Ground7/1 -> Pre-processor/1(Vzwp)
  Ground5/1 -> Pre-processor/3(mu_max)
  Ground/1 -> Pre-processor/8(alfa_f1)
  Ground1/1 -> Pre-processor/7(alfa_r1)
  Pre-processor/3(alfa_r) -> Terminator/1
  Pre-processor/1(Yaw_ref) -> Terminator2/1  "Yaw_ref"
  Ground3/1 -> Pre-processor/5(Fy_f)
  Ground6/1 -> Pre-processor/2(stuurhoek)
  Ground4/1 -> Pre-processor/4(a_zwpx)

== system generic_IsaacV3/CarMaker/IPG Vehicle/CarAndTrailer/CarAndTrailerUpd/CreateBus Brake.IF.In ==
  In : Inport
  BusCreator : BusCreator  Inputs=9
  Demux : Demux  Outputs=9
  Out : Outport
  wires:
  Demux/9 -> BusCreator/9  "Brake IF Trq_Reg RR"
  Demux/8 -> BusCreator/8  "Brake IF Trq_Reg RL"
  Demux/7 -> BusCreator/7  "Brake IF Trq_Reg FR"
  Demux/6 -> BusCreator/6  "Brake IF Trq_Reg FL"
  Demux/5 -> BusCreator/5  "Brake IF Trq_Reg_max RR"
  Demux/4 -> BusCreator/4  "Brake IF Trq_Reg_max RL"
  Demux/3 -> BusCreator/3  "Brake IF Trq_Reg_max FR"
  Demux/2 -> BusCreator/2  "Brake IF Trq_Reg_max FL"
  Demux/1 -> BusCreator/1  "Brake IF T_env"
  BusCreator/1 -> Out/1
  In/1 -> Demux/1

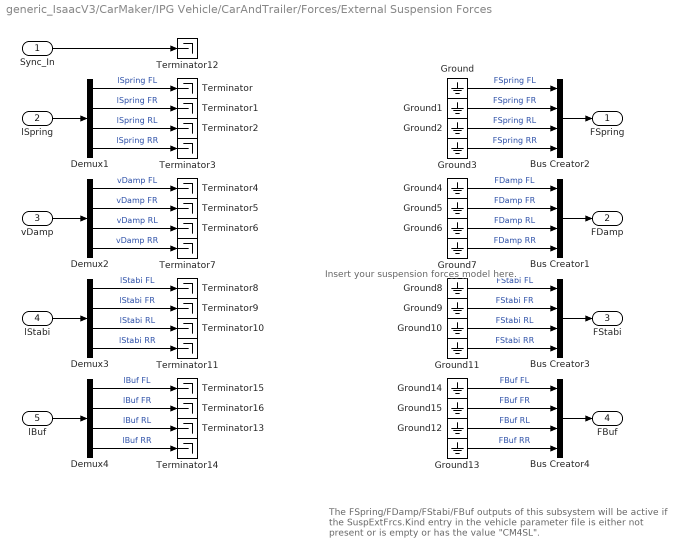
== system generic_IsaacV3/CarMaker/IPG Vehicle/CarAndTrailer/Forces/External Suspension Forces ==
  note: The FSpring/FDamp/FStabi/FBuf outputs of this subsystem will be
      | active if the SuspExtFrcs.Kind entry in the vehicle parameter file
      | is either not present or is empty or has the value "CM4SL".
  note: Insert your suspension forces model here.
  Sync_In : Inport
  lSpring : Inport  Port=2
  vDamp : Inport  Port=3
  lStabi : Inport  Port=4
  lBuf : Inport  Port=5
  Bus Creator{1..4} (4 alike) : BusCreator
  Demux{1..4} (4 alike) : Demux
  Ground{,1..15} (16 alike) : Ground
  Terminator{,1..16} (17 alike) : Terminator
  FSpring : Outport
  FDamp : Outport  Port=2
  FStabi : Outport  Port=3
  FBuf : Outport  Port=4
  wires:
  lBuf/1 -> Demux4/1
  Demux4/1 -> Terminator15/1  "lBuf FL"
  Demux4/2 -> Terminator16/1  "lBuf FR"
  Demux4/3 -> Terminator13/1  "lBuf RL"
  Demux4/4 -> Terminator14/1  "lBuf RR"
  Ground14/1 -> Bus Creator4/1  "FBuf FL"
  Ground15/1 -> Bus Creator4/2  "FBuf FR"
  Ground12/1 -> Bus Creator4/3  "FBuf RL"
  Ground13/1 -> Bus Creator4/4  "FBuf RR"
  Bus Creator4/1 -> FBuf/1
  Sync_In/1 -> Terminator12/1
  lSpring/1 -> Demux1/1
  vDamp/1 -> Demux2/1
  lStabi/1 -> Demux3/1
  Demux3/1 -> Terminator8/1  "lStabi FL"
  Demux3/2 -> Terminator9/1  "lStabi FR"
  Demux3/3 -> Terminator10/1  "lStabi RL"
  Demux3/4 -> Terminator11/1  "lStabi RR"
  Demux1/1 -> Terminator/1  "lSpring FL"
  Demux1/2 -> Terminator1/1  "lSpring FR"
  Demux1/3 -> Terminator2/1  "lSpring RL"
  Demux1/4 -> Terminator3/1  "lSpring RR"
  Demux2/1 -> Terminator4/1  "vDamp FL"
  Demux2/2 -> Terminator5/1  "vDamp FR"
  Demux2/3 -> Terminator6/1  "vDamp RL"
  Demux2/4 -> Terminator7/1  "vDamp RR"
  Bus Creator2/1 -> FSpring/1
  Ground/1 -> Bus Creator2/1  "FSpring FL"
  Ground1/1 -> Bus Creator2/2  "FSpring FR"
  Ground2/1 -> Bus Creator2/3  "FSpring RL"
  Ground3/1 -> Bus Creator2/4  "FSpring RR"
  Ground4/1 -> Bus Creator1/1  "FDamp FL"
  Ground5/1 -> Bus Creator1/2  "FDamp FR"
  Ground6/1 -> Bus Creator1/3  "FDamp RL"
  Ground7/1 -> Bus Creator1/4  "FDamp RR"
  Bus Creator1/1 -> FDamp/1
  Ground8/1 -> Bus Creator3/1  "FStabi FL"
  Ground9/1 -> Bus Creator3/2  "FStabi FR"
  Ground10/1 -> Bus Creator3/3  "FStabi RL"
  Ground11/1 -> Bus Creator3/4  "FStabi RR"
  Bus Creator3/1 -> FStabi/1

== system generic_IsaacV3/CarMaker/IPG Vehicle/CarAndTrailer/Forces/Tires ==
  note: The TireXX_Out signals will only be used if FileIdent is "CarMaker-Tire-CM4SL" in the tire parameter file!
      | An example parameter file can be found in Data/Tire/DT_CM4SL_UserTire.
  Sync_In : Inport
  TireFR_In : Inport  Port=2
  TireRL_In : Inport  Port=3
  TireRR_In : Inport  Port=4
  TireFL_In : Inport  Port=5
  Bus Creator{1..4} (4 alike) : BusCreator  Inputs=11
  Demux{1..3,8} (4 alike) : Demux  Outputs=7
  TireFL : Subsystem
  TireFR : Subsystem
  TireRL : Subsystem
  TireRR : Subsystem
  TireFR_Out : Outport
  TireRL_Out : Outport  Port=2
  TireRR_Out : Outport  Port=3
  TireFL_Out : Outport  Port=4
  wires:
  Sync_In/1 -> TireRR/1(Sync_In), TireRL/1(Sync_In), TireFR/1(Sync_In), TireFL/1(Sync_In)
  Bus Creator4/1 -> TireRR_Out/1
  Bus Creator2/1 -> TireRL_Out/1
  Bus Creator1/1 -> TireFR_Out/1
  Demux3/5 -> TireRR/6(Rim_turnv)  "Tire_In Rim_turnv"
  Demux3/4 -> TireRR/5(Rim_rotv)  "Tire_In Rim_rotv"
  Demux3/1 -> TireRR/2(Load)  "Tire_In Load"
  Demux3/7 -> TireRR/8(muRoad)  "Tire_In mu"
  Demux3/6 -> TireRR/7(InclinAngle)  "Tire_In Camber"
  Demux3/2 -> TireRR/3(vxtrans)  "Tire_In vxtrans"
  Demux3/3 -> TireRR/4(vytrans)  "Tire_In vytrans"
  TireRR/11(AlignTrq) -> Bus Creator4/11  "Tire_Out AlignTrq"
  TireRR/10(RollResist) -> Bus Creator4/10  "Tire_Out RollResist"
  TireRR/9(OverturnTrq) -> Bus Creator4/9  "Tire_Out OverturnTrq"
  TireRR/8(LoadFrc) -> Bus Creator4/8  "Tire_Out LoadFrc"
  TireRR/7(SideFrc) -> Bus Creator4/7  "Tire_Out SideFrc"
  TireRR/6(LongFrc) -> Bus Creator4/6  "Tire_Out LongFrc"
  TireRR/5(vBelt) -> Bus Creator4/5  "Tire_Out vBelt"
  TireRR/4(rBelt_eff) -> Bus Creator4/4  "Tire_Out rBelt_eff"
  TireRR/3(TurnSlp) -> Bus Creator4/3  "Tire_Out TurnSlp"
  TireRR/1(Slp) -> Bus Creator4/1  "Tire_Out Slp"
  TireRR/2(Alpha) -> Bus Creator4/2  "Tire_Out Alpha"
  Demux2/5 -> TireRL/6(Rim_turnv)  "Tire_In Rim_turnv"
  Demux2/4 -> TireRL/5(Rim_rotv)  "Tire_In Rim_rotv"
  Demux2/1 -> TireRL/2(Load)  "Tire_In Load"
  Demux2/7 -> TireRL/8(muRoad)  "Tire_In mu"
  Demux2/6 -> TireRL/7(InclinAngle)  "Tire_In Camber"
  Demux2/2 -> TireRL/3(vxtrans)  "Tire_In vxtrans"
  Demux2/3 -> TireRL/4(vytrans)  "Tire_In vytrans"
  TireRL/11(AlignTrq) -> Bus Creator2/11  "Tire_Out AlignTrq"
  TireRL/10(RollResist) -> Bus Creator2/10  "Tire_Out RollResist"
  TireRL/9(OverturnTrq) -> Bus Creator2/9  "Tire_Out OverturnTrq"
  TireRL/8(LoadFrc) -> Bus Creator2/8  "Tire_Out LoadFrc"
  TireRL/7(SideFrc) -> Bus Creator2/7  "Tire_Out SideFrc"
  TireRL/6(LongFrc) -> Bus Creator2/6  "Tire_Out LongFrc"
  TireRL/5(vBelt) -> Bus Creator2/5  "Tire_Out vBelt"
  TireRL/4(rBelt_eff) -> Bus Creator2/4  "Tire_Out rBelt_eff"
  TireRL/3(TurnSlp) -> Bus Creator2/3  "Tire_Out TurnSlp"
  TireRL/1(Slp) -> Bus Creator2/1  "Tire_Out Slp"
  TireRL/2(Alpha) -> Bus Creator2/2  "Tire_Out Alpha"
  Demux1/5 -> TireFR/6(Rim_turnv)  "Tire_In Rim_turnv"
  Demux1/4 -> TireFR/5(Rim_rotv)  "Tire_In Rim_rotv"
  Demux1/1 -> TireFR/2(Load)  "Tire_In Load"
  Demux1/7 -> TireFR/8(muRoad)  "Tire_In mu"
  Demux1/6 -> TireFR/7(InclinAngle)  "Tire_In Camber"
  Demux1/2 -> TireFR/3(vxtrans)  "Tire_In vxtrans"
  Demux1/3 -> TireFR/4(vytrans)  "Tire_In vytrans"
  TireFR/11(AlignTrq) -> Bus Creator1/11  "Tire_Out AlignTrq"
  TireFR/10(RollResist) -> Bus Creator1/10  "Tire_Out RollResist"
  TireFR/9(OverturnTrq) -> Bus Creator1/9  "Tire_Out OverturnTrq"
  TireFR/8(LoadFrc) -> Bus Creator1/8  "Tire_Out LoadFrc"
  TireFR/7(SideFrc) -> Bus Creator1/7  "Tire_Out SideFrc"
  TireFR/6(LongFrc) -> Bus Creator1/6  "Tire_Out LongFrc"
  TireFR/5(vBelt) -> Bus Creator1/5  "Tire_Out vBelt"
  TireFR/4(rBelt_eff) -> Bus Creator1/4  "Tire_Out rBelt_eff"
  TireFR/3(TurnSlp) -> Bus Creator1/3  "Tire_Out TurnSlp"
  TireFR/1(Slp) -> Bus Creator1/1  "Tire_Out Slp"
  TireFR/2(Alpha) -> Bus Creator1/2  "Tire_Out Alpha"
  Demux8/5 -> TireFL/6(Rim_turnv)  "Tire_In Rim_turnv"
  Demux8/4 -> TireFL/5(Rim_rotv)  "Tire_In Rim_rotv"
  TireFL_In/1 -> Demux8/1
  Demux8/1 -> TireFL/2(Load)  "Tire_In Load"
  Demux8/7 -> TireFL/8(muRoad)  "Tire_In mu"
  Demux8/6 -> TireFL/7(InclinAngle)  "Tire_In Camber"
  Demux8/2 -> TireFL/3(vxtrans)  "Tire_In vxtrans"
  Demux8/3 -> TireFL/4(vytrans)  "Tire_In vytrans"
  TireFL/11(AlignTrq) -> Bus Creator3/11  "Tire_Out AlignTrq"
  TireFL/10(RollResist) -> Bus Creator3/10  "Tire_Out RollResist"
  TireFL/9(OverturnTrq) -> Bus Creator3/9  "Tire_Out OverturnTrq"
  TireFL/8(LoadFrc) -> Bus Creator3/8  "Tire_Out LoadFrc"
  TireFL/7(SideFrc) -> Bus Creator3/7  "Tire_Out SideFrc"
  TireFL/6(LongFrc) -> Bus Creator3/6  "Tire_Out LongFrc"
  TireFL/5(vBelt) -> Bus Creator3/5  "Tire_Out vBelt"
  TireFL/4(rBelt_eff) -> Bus Creator3/4  "Tire_Out rBelt_eff"
  TireFL/3(TurnSlp) -> Bus Creator3/3  "Tire_Out TurnSlp"
  TireFL/1(Slp) -> Bus Creator3/1  "Tire_Out Slp"
  TireFL/2(Alpha) -> Bus Creator3/2  "Tire_Out Alpha"
  Bus Creator3/1 -> TireFL_Out/1
  TireFR_In/1 -> Demux1/1
  TireRL_In/1 -> Demux2/1
  TireRR_In/1 -> Demux3/1

== system generic_IsaacV3/CarMaker/IPG Vehicle/CarAndTrailer/Forces/Vehicle Forces ==
  Sync_In : Inport
  Bus Creator1 : BusCreator  Inputs=12
  Bus Creator5 : BusCreator  Inputs=13
  Bus Creator8 : BusCreator  Inputs=16
  Demux : Demux  Outputs=16
  Demux1 : Demux  Outputs=12
  Demux5 : Demux  Outputs=13
  Forces : S-Function  FunctionName=CM_Sfun  Parameters='Forces'
  Sync_Out : Outport
  Car.Virtual : Outport  Port=2
  Car.Aero : Outport  Port=3
  Car.Load : Outport  Port=4
  wires:
  Demux/16 -> Bus Creator8/16  "Car Load_3 tz"
  Demux/15 -> Bus Creator8/15  "Car Load_3 ty"
  Demux/14 -> Bus Creator8/14  "Car Load_3 tx"
  Demux/13 -> Bus Creator8/13  "Car Load_3 mass"
  Demux1/12 -> Bus Creator1/12  "Car Virtual Trq_0 z"
  Demux1/11 -> Bus Creator1/11  "Car Virtual Trq_0 y"
  Demux1/10 -> Bus Creator1/10  "Car Virtual Trq_0 x"
  Demux1/9 -> Bus Creator1/9  "Car Virtual Trq_1 z"
  Demux1/8 -> Bus Creator1/8  "Car Virtual Trq_1 y"
  Demux1/7 -> Bus Creator1/7  "Car Virtual Trq_1 x"
  Demux1/6 -> Bus Creator1/6  "Car Virtual Frc_0 z"
  Demux1/5 -> Bus Creator1/5  "Car Virtual Frc_0 y"
  Demux1/4 -> Bus Creator1/4  "Car Virtual Frc_0 x"
  Sync_In/1 -> Forces/1
  Forces/1 -> Sync_Out/1
  Bus Creator5/1 -> Car.Aero/1
  Demux1/1 -> Bus Creator1/1  "Car Virtual Frc_1 x"
  Demux1/2 -> Bus Creator1/2  "Car Virtual Frc_1 y"
  Demux1/3 -> Bus Creator1/3  "Car Virtual Frc_1 z"
  Forces/3 -> Demux5/1
  Forces/2 -> Demux1/1
  Bus Creator1/1 -> Car.Virtual/1
  Bus Creator8/1 -> Car.Load/1
  Demux/1 -> Bus Creator8/1  "Car Load_0 mass"
  Demux/2 -> Bus Creator8/2  "Car Load_0 tx"
  Demux/3 -> Bus Creator8/3  "Car Load_0 ty"
  Demux/4 -> Bus Creator8/4  "Car Load_0 tz"
  Demux/5 -> Bus Creator8/5  "Car Load_1 mass"
  Demux/6 -> Bus Creator8/6  "Car Load_1 tx"
  Demux/7 -> Bus Creator8/7  "Car Load_1 ty"
  Demux/8 -> Bus Creator8/8  "Car Load_1 tz"
  Demux/9 -> Bus Creator8/9  "Car Load_2 mass"
  Demux/10 -> Bus Creator8/10  "Car Load_2 tx"
  Demux/11 -> Bus Creator8/11  "Car Load_2 ty"
  Demux/12 -> Bus Creator8/12  "Car Load_2 tz"
  Forces/4 -> Demux/1
  Demux5/11 -> Bus Creator5/11  "car Aero Trq_1 x"
  Demux5/12 -> Bus Creator5/12  "car Aero Trq_1 y"
  Demux5/13 -> Bus Creator5/13  "car Aero Trq_1 z"
  Demux5/10 -> Bus Creator5/10  "car Aero Frc_1 z"
  Demux5/9 -> Bus Creator5/9  "car Aero Frc_1 y"
  Demux5/8 -> Bus Creator5/8  "car Aero Frc_1 x"
  Demux5/1 -> Bus Creator5/1  "Vehicle sRoadAero"
  Demux5/2 -> Bus Creator5/2  "Vehicle Wind_vel_0 x"
  Demux5/3 -> Bus Creator5/3  "Vehicle Wind_vel_0 y"
  Demux5/4 -> Bus Creator5/4  "Vehicle Wind_vel_0 z"
  Demux5/5 -> Bus Creator5/5  "car Aero vRes_1 x"
  Demux5/6 -> Bus Creator5/6  "car Aero vRes_1 y"
  Demux5/7 -> Bus Creator5/7  "car Aero vRes_1 z"

== system generic_IsaacV3/CarMaker/IPG Vehicle/CarAndTrailer/Trailer/CreateBus Car.Hitch.FrcTrq ==
  In1 : Inport
  Bus Creator7 : BusCreator  Inputs=6
  Demux7 : Demux  Outputs=6
  Car.Hitch.FrcTrq : Outport
  wires:
  In1/1 -> Demux7/1
  Bus Creator7/1 -> Car.Hitch.FrcTrq/1
  Demux7/6 -> Bus Creator7/6  "Car Hitch Trq2Car z"
  Demux7/5 -> Bus Creator7/5  "Car Hitch Trq2Car y"
  Demux7/4 -> Bus Creator7/4  "Car Hitch Trq2Car x"
  Demux7/3 -> Bus Creator7/3  "Car Hitch Frc2Car z"
  Demux7/2 -> Bus Creator7/2  "Car Hitch Frc2Car y"
  Demux7/1 -> Bus Creator7/1  "Car Hitch Frc2Car x"

== system generic_IsaacV3/CarMaker/IPG Vehicle/CarAndTrailer/Trailer/CreateBus Vhcl.Motion ==
  In1 : Inport
  Demux1 : Demux  Outputs=16
  Mux1 : Mux  Inputs=16
  Out1 : Outport
  wires:
  Demux1/1 -> Mux1/1  "Vhcl v"
  Demux1/2 -> Mux1/2  "Vhcl Distance"
  Demux1/3 -> Mux1/3  "Vhcl sRoad"
  Demux1/4 -> Mux1/4  "Vhcl sRoadAero"
  Demux1/5 -> Mux1/5  "Vhcl Hitch_Pos x"
  Demux1/6 -> Mux1/6  "Vhcl Hitch_Pos y"
  Demux1/7 -> Mux1/7  "Vhcl Hitch_Pos z"
  Demux1/8 -> Mux1/8  "Vhcl Roll"
  Demux1/9 -> Mux1/9  "Vhcl RollVel"
  Demux1/10 -> Mux1/10  "Vhcl RollAcc"
  Demux1/11 -> Mux1/11  "Vhcl Pitch"
  Demux1/12 -> Mux1/12  "Vhcl PitchVel"
  Demux1/13 -> Mux1/13  "Vhcl PitchAcc"
  Demux1/14 -> Mux1/14  "Vhcl Yaw"
  Demux1/15 -> Mux1/15  "Vhcl YawRate"
  Demux1/16 -> Mux1/16  "Vhcl YawAcc"
  In1/1 -> Demux1/1
  Mux1/1 -> Out1/1

== system generic_IsaacV3/CarMaker/IPG Vehicle/CarAndTrailer/Trailer/CreateBus Vhcl.PoI ==
  In1 : Inport
  Bus Creator3 : BusCreator  Inputs=18
  Demux3 : Demux  Outputs=18
  Out1 : Outport
  wires:
  Demux3/18 -> Bus Creator3/18  "Vhcl PoI_GCS Elev"
  Demux3/17 -> Bus Creator3/17  "Vhcl PoI_GCS Lat"
  Demux3/16 -> Bus Creator3/16  "Vhcl PoI_GCS Long"
  Demux3/15 -> Bus Creator3/15  "Vhcl PoI_Acc_1 z"
  Demux3/14 -> Bus Creator3/14  "Vhcl PoI_Acc_1 y"
  Demux3/13 -> Bus Creator3/13  "Vhcl PoI_Acc_1 x"
  Demux3/12 -> Bus Creator3/12  "Vhcl PoI_Vel_1 z"
  Demux3/11 -> Bus Creator3/11  "Vhcl PoI_Vel_1 y"
  Demux3/10 -> Bus Creator3/10  "Vhcl PoI_Vel_1 x"
  Demux3/9 -> Bus Creator3/9  "Vhcl PoI_Acc z"
  Demux3/8 -> Bus Creator3/8  "Vhcl PoI_Acc y"
  Demux3/7 -> Bus Creator3/7  "Vhcl PoI_Acc x"
  Demux3/6 -> Bus Creator3/6  "Vhcl PoI_Vel z"
  Demux3/5 -> Bus Creator3/5  "Vhcl PoI_Vel y"
  Demux3/4 -> Bus Creator3/4  "Vhcl PoI_Vel x"
  Demux3/3 -> Bus Creator3/3  "Vhcl PoI_Pos z"
  Demux3/2 -> Bus Creator3/2  "Vhcl PoI_Pos y"
  In1/1 -> Demux3/1
  Bus Creator3/1 -> Out1/1
  Demux3/1 -> Bus Creator3/1  "Vhcl PoI_Pos x"

== system generic_IsaacV3/CarMaker/IPG Vehicle/CarAndTrailer/Trailer/CreateBus Vhcl.Steering ==
  In1 : Inport
  Bus Creator3 : BusCreator
  Demux : Demux
  Out1 : Outport
  wires:
  Bus Creator3/1 -> Out1/1
  Demux/1 -> Bus Creator3/1  "Vhcl Steering Ang"
  Demux/3 -> Bus Creator3/3  "Vhcl Steering AngAcc"
  Demux/2 -> Bus Creator3/2  "Vhcl Steering AngVel"
  Demux/4 -> Bus Creator3/4  "Vhcl Steering Trq"
  In1/1 -> Demux/1

== system generic_IsaacV3/CarMaker/IPG Vehicle/CarAndTrailer/Trailer/CreateBus Vhcl.Wheel.FL ==
  In1 : Inport
  Bus Creator3 : BusCreator  Inputs=14
  Demux3 : Demux  Outputs=14
  Out1 : Outport
  wires:
  Demux3/14 -> Bus Creator3/14  "Vhcl Wheel FL Trq_WhlBearing"
  Demux3/13 -> Bus Creator3/13  "Vhcl Wheel FL Trq_T2W"
  Demux3/12 -> Bus Creator3/12  "Vhcl Wheel FL SideSlip"
  Demux3/11 -> Bus Creator3/11  "Vhcl Wheel FL LongSlip"
  Demux3/10 -> Bus Creator3/10  "Vhcl Wheel FL vBelt"
  Demux3/9 -> Bus Creator3/9  "Vhcl Wheel FL Fz"
  Demux3/8 -> Bus Creator3/8  "Vhcl Wheel FL Fy"
  Demux3/7 -> Bus Creator3/7  "Vhcl Wheel FL Fx"
  Demux3/6 -> Bus Creator3/6  "Vhcl Wheel FL r_zxy z"
  Demux3/5 -> Bus Creator3/5  "Vhcl Wheel FL r_zxy y"
  Demux3/4 -> Bus Creator3/4  "Vhcl Wheel FL r_zxy x"
  Demux3/3 -> Bus Creator3/3  "Vhcl Wheel FL t z"
  Demux3/2 -> Bus Creator3/2  "Vhcl Wheel FL t y"
  In1/1 -> Demux3/1
  Bus Creator3/1 -> Out1/1
  Demux3/1 -> Bus Creator3/1  "Vhcl Wheel FL t x"
